simulink model "NeuromuscularModel"  (R2019b)
settings: Solver=ode15s  StartTime=0.0  StopTime=inf  MaxStep=.01  RelTol=1e-4  AbsTol=1e-6  EnableMultiTasking=on
values from neighbouring files (symbols this model uses):
  LceOffsetTA = 1-0.5*w    [ControlParams2.m]
  legLengthClr = .9    (= 0.9)    [ControlParams2.m]    (also in assignGains.m = Gains(20); assignGains2.m = Gains(20); assignGainsSagittal.m = GainsSagittal(39))
  LongDelay = 0.020    (= 0.02)    [ControlParams2.m]
  MidDelay = 0.010    (= 0.01)    [ControlParams2.m]
  N = 82    [vcmaes_1.5cm_0.9ms_Umb10_kneelim1_mstoptorque2.mat]
  ShortDelay = 0.005    [ControlParams2.m]
  simbiconGainD = 5*pi/180    (= 0.0872664625997)    [ControlParams2.m]    (also in assignGains.m = Gains(21); assignGains2.m = Gains(21); assignGainsSagittal.m = GainsSagittal(41))
  simbiconGainDAbd = 0.1421    [ControlParams2.m]    (also in assignGains.m = Gains(33))
  simbiconGainV = 5*pi/180    (= 0.0872664625997)    [ControlParams2.m]    (also in assignGains.m = Gains(22); assignGains2.m = Gains(22); assignGainsSagittal.m = GainsSagittal(42))
  simbiconGainVAbd = 0.2148    [ControlParams2.m]    (also in assignGains.m = Gains(34))
  simbiconLegAngle0 = 85*pi/180    (= 1.4835298642)    [ControlParams2.m]    (also in assignGains.m = Gains(23); assignGains2.m = Gains(23); assignGainsSagittal.m = GainsSagittal(40))
  simbiconLegAngle0Abd = -0.0133    [ControlParams2.m]    (also in assignGains.m = Gains(32))
undefined symbols (not defined in the file or in its folder): footCenterToCGDist, footInertia, footMass, g, hatHipToCenterDistLen, loptGAS, loptTA, lslackGAS, magnitude, phimaxGASa, phimaxGASk, phirefGASa, phirefGASk, rGASa, rGASk, rhoGASa, rhoGASk, X, Y, Z
libraries: NeuroMuscularLibrary x101, nesl_utility x30, sm_lib x21, simulink x4, simulink_extras x2, NeuroMuscularLibrary2 x2
(part 3 of 3)

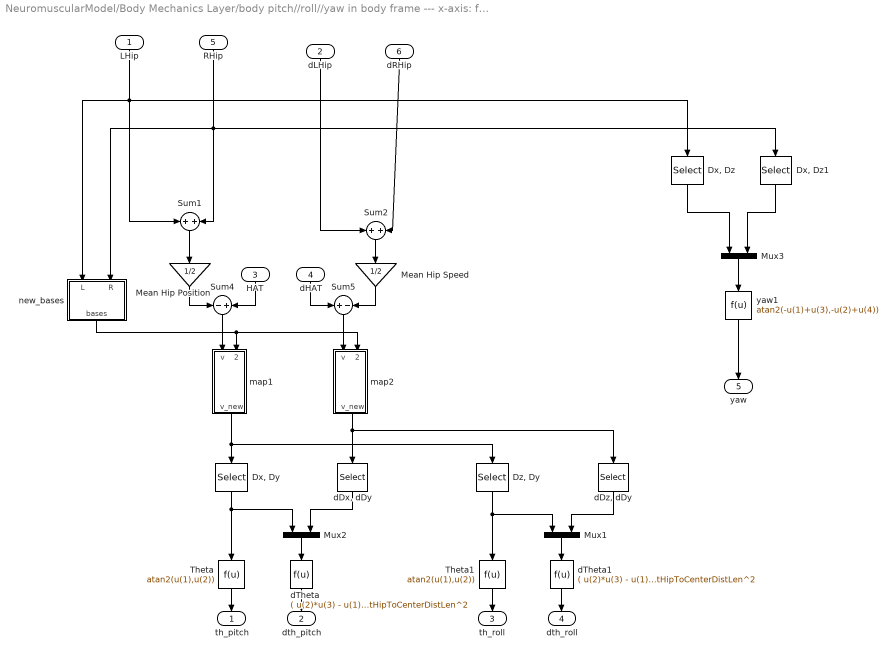
== system NeuromuscularModel/Body Mechanics Layer/body pitch//roll//yaw in body frame --- x-axis: forward y-axis: leftward z-axis: parallel to gravity ==
  LHip : Inport
  dLHip : Inport  Port=2
  HAT : Inport  Port=3
  dHAT : Inport  Port=4
  RHip : Inport  Port=5
  dRHip : Inport  Port=6
  " Mean Hip Speed" : Gain  Gain=1/2
  "Dx, Dy" : Selector  InputPortWidth=3  IndexOptions=Index vector (dialog)  Indices=[1 2]  OutputSizes=1
  "Dx, Dz" : Selector  InputPortWidth=3  IndexOptions=Index vector (dialog)  Indices=[1 3]  OutputSizes=1
  "Dx, Dz1" : Selector  InputPortWidth=3  IndexOptions=Index vector (dialog)  Indices=[1 3]  OutputSizes=1
  "Dz, Dy" : Selector  InputPortWidth=3  IndexOptions=Index vector (dialog)  Indices=[3 2]  OutputSizes=1
  Mean Hip Position : Gain  Gain=1/2
  Mux1 : Mux  Inputs=2
  Mux2 : Mux  Inputs=2
  Mux3 : Mux  Inputs=2
  Sum1 : Sum
  Sum2 : Sum
  Sum4 : Sum  Inputs=-+
  Sum5 : Sum  Inputs=+-
  Theta : Fcn  Expr=atan2(u(1),u(2))
  Theta1 : Fcn  Expr=atan2(u(1),u(2))
  "dDx, dDy" : Selector  InputPortWidth=3  IndexOptions=Index vector (dialog)  Indices=[1 2]  OutputSizes=1
  "dDz, dDy" : Selector  InputPortWidth=3  IndexOptions=Index vector (dialog)  Indices=[3 2]  OutputSizes=1
  dTheta : Fcn  Expr=( u(2)*u(3) - u(1)*u(4) ) / hatHipToCenterDistLen^2
  dTheta1 : Fcn  Expr=( u(2)*u(3) - u(1)*u(4) ) / hatHipToCenterDistLen^2
  map1 : Subsystem
  map2 : Subsystem
  new_bases : Subsystem
  yaw1 : Fcn  Expr=atan2(-u(1)+u(3),-u(2)+u(4))
  th_pitch : Outport
  dth_pitch : Outport  Port=2
  th_roll : Outport  Port=3
  dth_roll : Outport  Port=4
  yaw : Outport  Port=5
  wires:
  dHAT/1 -> Sum5/1
  "dDx, dDy"/1 -> Mux2/2
  Mux2/1 -> dTheta/1
  Sum1/1 -> Mean Hip Position/1
  Sum2/1 -> " Mean Hip Speed"/1
  HAT/1 -> Sum4/2
  Mean Hip Position/1 -> Sum4/1
  " Mean Hip Speed"/1 -> Sum5/2
  "Dx, Dy"/1 -> Mux2/1, Theta/1
  LHip/1 -> Sum1/1, new_bases/1(L), "Dx, Dz"/1
  RHip/1 -> Sum1/2, new_bases/2(R), "Dx, Dz1"/1
  dLHip/1 -> Sum2/1
  dRHip/1 -> Sum2/2
  Theta/1 -> th_pitch/1
  dTheta/1 -> dth_pitch/1
  Sum4/1 -> map1/1(v)
  map1/1(v_new) -> "Dx, Dy"/1, "Dz, Dy"/1
  new_bases/1(bases) -> map1/2(basis), map2/2(basis)
  Sum5/1 -> map2/1(v)
  map2/1(v_new) -> "dDx, dDy"/1, "dDz, dDy"/1
  "dDz, dDy"/1 -> Mux1/2
  Mux1/1 -> dTheta1/1
  "Dz, Dy"/1 -> Mux1/1, Theta1/1
  Theta1/1 -> th_roll/1
  dTheta1/1 -> dth_roll/1
  "Dx, Dz"/1 -> Mux3/1
  "Dx, Dz1"/1 -> Mux3/2
  Mux3/1 -> yaw1/1
  yaw1/1 -> yaw/1

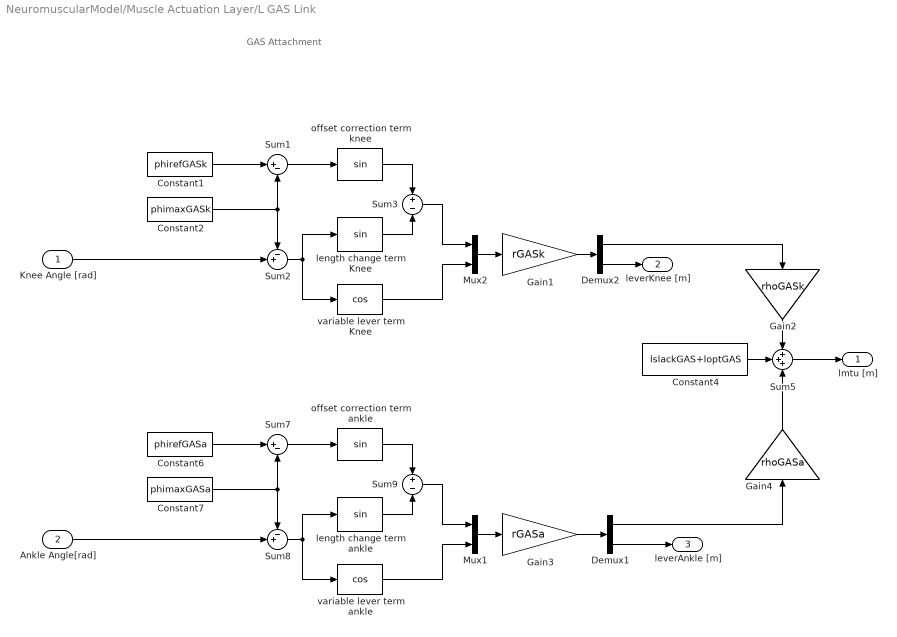
== system NeuromuscularModel/Muscle Actuation Layer/L GAS Link ==
  note: GAS Attachment
  Knee Angle [rad] : Inport
  Ankle Angle[rad] : Inport  Port=2
  Constant1 : Constant  Value=phirefGASk
  Constant2 : Constant  Value=phimaxGASk
  Constant4 : Constant  Value=lslackGAS+loptGAS
  Constant6 : Constant  Value=phirefGASa
  Constant7 : Constant  Value=phimaxGASa
  Demux1 : Demux  Outputs=2
  Demux2 : Demux  Outputs=2
  Gain1 : Gain  Gain=rGASk
  Gain2 : Gain  Gain=rhoGASk
  Gain3 : Gain  Gain=rGASa
  Gain4 : Gain  Gain=rhoGASa
  Mux1 : Mux  Inputs=2
  Mux2 : Mux  Inputs=2
  Sum1 : Sum  Inputs=|+-
  Sum2 : Sum  Inputs=-+|
  Sum3 : Sum  Inputs=+-
  Sum5 : Sum  Inputs=+++
  Sum7 : Sum  Inputs=|+-
  Sum8 : Sum  Inputs=-+|
  Sum9 : Sum  Inputs=+-
  length change term Knee : Trigonometry
  length change term ankle : Trigonometry
  offset correction term ankle : Trigonometry
  offset correction term knee : Trigonometry
  variable lever term Knee : Trigonometry  Operator=cos
  variable lever term ankle : Trigonometry  Operator=cos
  lmtu [m] : Outport
  leverKnee [m] : Outport  Port=2
  leverAnkle [m] : Outport  Port=3
  wires:
  Ankle Angle[rad]/1 -> Sum8/2
  Sum5/1 -> lmtu [m]/1
  variable lever term ankle/1 -> Mux1/2
  Demux1/2 -> leverAnkle [m]/1
  Sum8/1 -> variable lever term ankle/1, length change term ankle/1
  Constant7/1 -> Sum8/1, Sum7/2
  Sum7/1 -> offset correction term ankle/1
  Constant6/1 -> Sum7/1
  length change term ankle/1 -> Sum9/2
  offset correction term ankle/1 -> Sum9/1
  Sum9/1 -> Mux1/1
  Constant4/1 -> Sum5/2
  Mux1/1 -> Gain3/1
  Gain3/1 -> Demux1/1
  Demux1/1 -> Gain4/1
  Gain4/1 -> Sum5/3
  Knee Angle [rad]/1 -> Sum2/2
  variable lever term Knee/1 -> Mux2/2
  Sum2/1 -> variable lever term Knee/1, length change term Knee/1
  Constant2/1 -> Sum2/1, Sum1/2
  Sum1/1 -> offset correction term knee/1
  Constant1/1 -> Sum1/1
  length change term Knee/1 -> Sum3/2
  offset correction term knee/1 -> Sum3/1
  Sum3/1 -> Mux2/1
  Mux2/1 -> Gain1/1
  Gain1/1 -> Demux2/1
  Demux2/2 -> leverKnee [m]/1
  Demux2/1 -> Gain2/1
  Gain2/1 -> Sum5/1

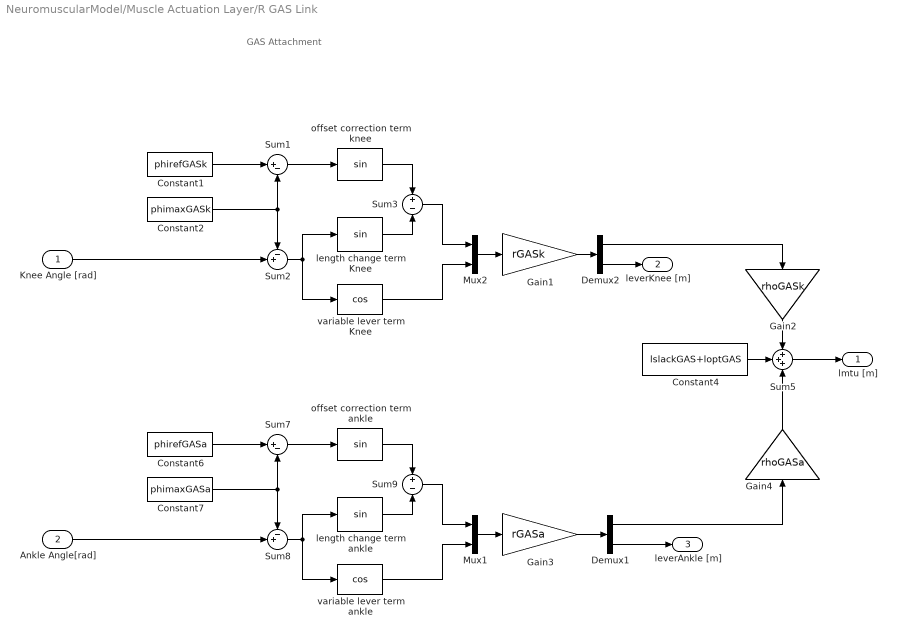
== system NeuromuscularModel/Muscle Actuation Layer/R GAS Link ==
  note: GAS Attachment
  Knee Angle [rad] : Inport
  Ankle Angle[rad] : Inport  Port=2
  Constant1 : Constant  Value=phirefGASk
  Constant2 : Constant  Value=phimaxGASk
  Constant4 : Constant  Value=lslackGAS+loptGAS
  Constant6 : Constant  Value=phirefGASa
  Constant7 : Constant  Value=phimaxGASa
  Demux1 : Demux  Outputs=2
  Demux2 : Demux  Outputs=2
  Gain1 : Gain  Gain=rGASk
  Gain2 : Gain  Gain=rhoGASk
  Gain3 : Gain  Gain=rGASa
  Gain4 : Gain  Gain=rhoGASa
  Mux1 : Mux  Inputs=2
  Mux2 : Mux  Inputs=2
  Sum1 : Sum  Inputs=|+-
  Sum2 : Sum  Inputs=-+|
  Sum3 : Sum  Inputs=+-
  Sum5 : Sum  Inputs=+++
  Sum7 : Sum  Inputs=|+-
  Sum8 : Sum  Inputs=-+|
  Sum9 : Sum  Inputs=+-
  length change term Knee : Trigonometry
  length change term ankle : Trigonometry
  offset correction term ankle : Trigonometry
  offset correction term knee : Trigonometry
  variable lever term Knee : Trigonometry  Operator=cos
  variable lever term ankle : Trigonometry  Operator=cos
  lmtu [m] : Outport
  leverKnee [m] : Outport  Port=2
  leverAnkle [m] : Outport  Port=3
  wires:
  Ankle Angle[rad]/1 -> Sum8/2
  Sum5/1 -> lmtu [m]/1
  variable lever term ankle/1 -> Mux1/2
  Demux1/2 -> leverAnkle [m]/1
  Sum8/1 -> variable lever term ankle/1, length change term ankle/1
  Constant7/1 -> Sum8/1, Sum7/2
  Sum7/1 -> offset correction term ankle/1
  Constant6/1 -> Sum7/1
  length change term ankle/1 -> Sum9/2
  offset correction term ankle/1 -> Sum9/1
  Sum9/1 -> Mux1/1
  Constant4/1 -> Sum5/2
  Mux1/1 -> Gain3/1
  Gain3/1 -> Demux1/1
  Demux1/1 -> Gain4/1
  Gain4/1 -> Sum5/3
  Knee Angle [rad]/1 -> Sum2/2
  variable lever term Knee/1 -> Mux2/2
  Sum2/1 -> variable lever term Knee/1, length change term Knee/1
  Constant2/1 -> Sum2/1, Sum1/2
  Sum1/1 -> offset correction term knee/1
  Constant1/1 -> Sum1/1
  length change term Knee/1 -> Sum3/2
  offset correction term knee/1 -> Sum3/1
  Sum3/1 -> Mux2/1
  Mux2/1 -> Gain1/1
  Gain1/1 -> Demux2/1
  Demux2/2 -> leverKnee [m]/1
  Demux2/1 -> Gain2/1
  Gain2/1 -> Sum5/1

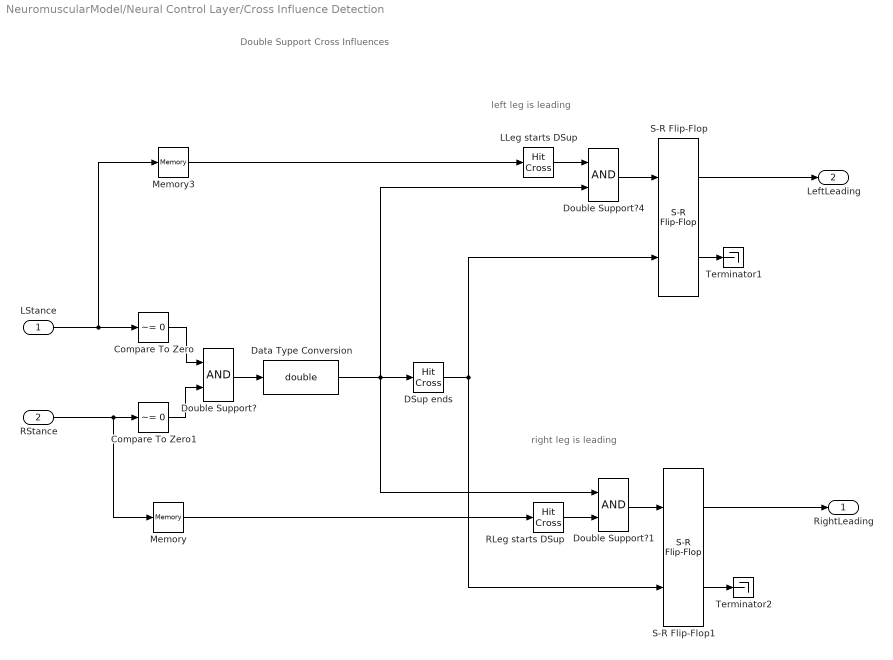
== system NeuromuscularModel/Neural Control Layer/Cross Influence Detection ==
  note: right leg is leading
  note: left leg is leading
  note: Double Support Cross Influences
  LStance : Inport
  RStance : Inport  Port=2
  Compare To Zero : simulink/Logic and Bit Operations/Compare To Zero  relop=~=  OutDataTypeStr=boolean
  Compare To Zero1 : simulink/Logic and Bit Operations/Compare To Zero  relop=~=  OutDataTypeStr=boolean
  DSup ends : HitCross  HitCrossingOffset=0.5  HitCrossingDirection=falling  ZeroCross=off
  Data Type Conversion : DataTypeConversion  OutDataTypeStr=double
  Double Support? : Logic  AllPortsSameDT=off
  Double Support?1 : Logic  AllPortsSameDT=off
  Double Support?4 : Logic  AllPortsSameDT=off
  LLeg starts DSup : HitCross  HitCrossingOffset=0.5  HitCrossingDirection=rising  ZeroCross=off
  Memory : Memory
  Memory3 : Memory
  RLeg starts DSup : HitCross  HitCrossingOffset=0.5  HitCrossingDirection=rising  ZeroCross=off
  S-R Flip-Flop : simulink_extras/Flip Flops/S-R Flip-Flop  initial_condition=0
  S-R Flip-Flop1 : simulink_extras/Flip Flops/S-R Flip-Flop  initial_condition=0
  Terminator1 : Terminator
  Terminator2 : Terminator
  RightLeading : Outport
  LeftLeading : Outport  Port=2
  wires:
  S-R Flip-Flop/2 -> Terminator1/1
  S-R Flip-Flop/1 -> LeftLeading/1
  S-R Flip-Flop1/2 -> Terminator2/1
  LStance/1 -> Memory3/1, Compare To Zero/1
  RStance/1 -> Compare To Zero1/1, Memory/1
  S-R Flip-Flop1/1 -> RightLeading/1
  Memory/1 -> RLeg starts DSup/1
  RLeg starts DSup/1 -> Double Support?1/2
  Double Support?1/1 -> S-R Flip-Flop1/1
  Memory3/1 -> LLeg starts DSup/1
  LLeg starts DSup/1 -> Double Support?4/1
  Double Support?4/1 -> S-R Flip-Flop/1
  DSup ends/1 -> S-R Flip-Flop/2, S-R Flip-Flop1/2
  Compare To Zero/1 -> Double Support?/1
  Compare To Zero1/1 -> Double Support?/2
  Double Support?/1 -> Data Type Conversion/1
  Data Type Conversion/1 -> Double Support?1/1, Double Support?4/2, DSup ends/1

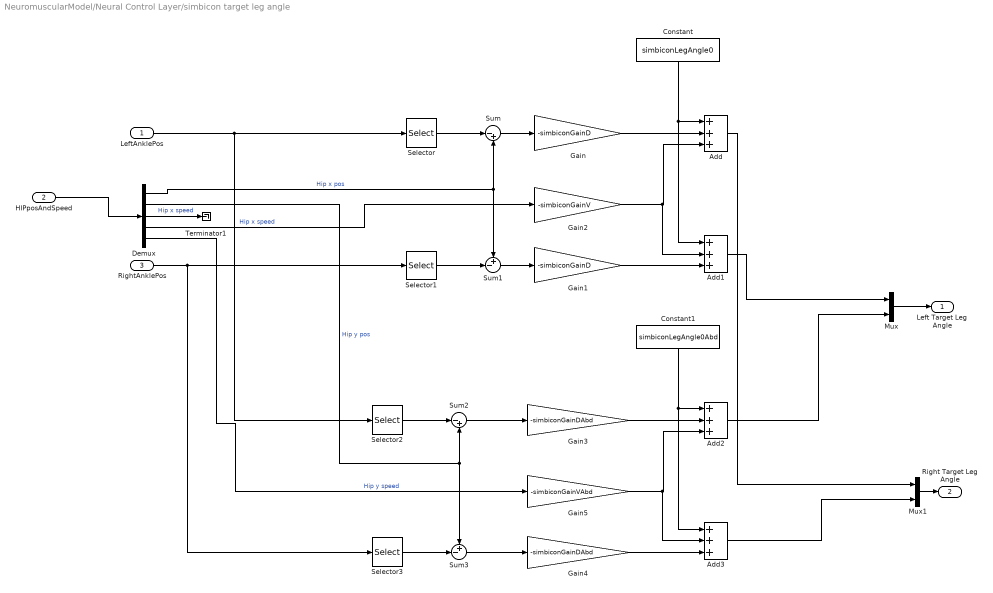
== system NeuromuscularModel/Neural Control Layer/simbicon target leg angle ==
  LeftAnklePos : Inport
  HIPposAndSpeed : Inport  Port=2
  RightAnklePos : Inport  Port=3
  Add{,1..3} (4 alike) : Sum  Inputs=+++
  Constant : Constant  Value=simbiconLegAngle0
  Constant1 : Constant  Value=simbiconLegAngle0Abd
  Demux : Demux  Outputs=5
  Gain : Gain  Gain=-simbiconGainD
  Gain1 : Gain  Gain=-simbiconGainD
  Gain2 : Gain  Gain=-simbiconGainV
  Gain3 : Gain  Gain=-simbiconGainDAbd
  Gain4 : Gain  Gain=-simbiconGainDAbd
  Gain5 : Gain  Gain=-simbiconGainVAbd
  Mux : Mux  Inputs=2
  Mux1 : Mux  Inputs=2
  Selector : Selector  InputPortWidth=3  IndexOptions=Index vector (dialog)  Indices=[1]  OutputSizes=1
  Selector1 : Selector  InputPortWidth=3  IndexOptions=Index vector (dialog)  Indices=[1]  OutputSizes=1
  Selector2 : Selector  InputPortWidth=3  IndexOptions=Index vector (dialog)  Indices=[3]  OutputSizes=1
  Selector3 : Selector  InputPortWidth=3  IndexOptions=Index vector (dialog)  Indices=3  OutputSizes=1
  Sum : Sum  Inputs=|-+
  Sum1 : Sum  Inputs=+-|
  Sum2 : Sum  Inputs=|-+
  Sum3 : Sum  Inputs=+-|
  Terminator1 : Terminator
  Left Target Leg Angle : Outport
  Right Target Leg Angle : Outport  Port=2
  wires:
  HIPposAndSpeed/1 -> Demux/1
  Demux/1 -> Sum/2, Sum1/1  "Hip x pos"
  Sum/1 -> Gain/1
  Sum1/1 -> Gain1/1
  Gain/1 -> Add/2
  Gain2/1 -> Add1/2, Add/3
  Gain1/1 -> Add1/3
  Constant/1 -> Add/1, Add1/1
  LeftAnklePos/1 -> Selector2/1, Selector/1
  Selector/1 -> Sum/1
  RightAnklePos/1 -> Selector3/1, Selector1/1
  Selector1/1 -> Sum1/2
  Demux/2 -> Sum2/2, Sum3/1  "Hip y pos"
  Selector3/1 -> Sum3/2
  Gain5/1 -> Add3/2, Add2/3
  Selector2/1 -> Sum2/1
  Gain4/1 -> Add3/3
  Sum2/1 -> Gain3/1
  Gain3/1 -> Add2/2
  Sum3/1 -> Gain4/1
  Constant1/1 -> Add2/1, Add3/1
  Demux/4 -> Gain2/1  "Hip x speed"
  Demux/5 -> Gain5/1  "Hip y speed"
  Demux/3 -> Terminator1/1  "Hip x speed"
  Add1/1 -> Mux/1
  Add2/1 -> Mux/2
  Add3/1 -> Mux1/2
  Add/1 -> Mux1/1
  Mux1/1 -> Right Target Leg Angle/1
  Mux/1 -> Left Target Leg Angle/1

== system NeuromuscularModel/Body Mechanics Layer/body pitch//roll//yaw in body frame --- x-axis: forward y-axis: leftward z-axis: parallel to gravity/map1 ==
  v : Inport
  basis : Inport  Port=2
  Demux : Demux  Outputs=3
  Dot Product : DotProduct  InputSameDT=on  OutDataTypeStr=Inherit: Inherit via internal rule
  Dot Product1 : DotProduct  InputSameDT=on  OutDataTypeStr=Inherit: Inherit via internal rule
  Dot Product2 : DotProduct  InputSameDT=on  OutDataTypeStr=Inherit: Inherit via internal rule
  Mux3 : Mux  Inputs=3
  v_new : Outport
  wires:
  v/1 -> Dot Product2/2, Dot Product1/2, Dot Product/2
  Dot Product/1 -> Mux3/1
  Dot Product1/1 -> Mux3/2
  Dot Product2/1 -> Mux3/3
  Mux3/1 -> v_new/1  "v1"
  basis/1 -> Demux/1
  Demux/1 -> Dot Product/1
  Demux/2 -> Dot Product1/1
  Demux/3 -> Dot Product2/1

== system NeuromuscularModel/Body Mechanics Layer/body pitch//roll//yaw in body frame --- x-axis: forward y-axis: leftward z-axis: parallel to gravity/map2 ==
  v : Inport
  basis : Inport  Port=2
  Demux : Demux  Outputs=3
  Dot Product : DotProduct  InputSameDT=on  OutDataTypeStr=Inherit: Inherit via internal rule
  Dot Product1 : DotProduct  InputSameDT=on  OutDataTypeStr=Inherit: Inherit via internal rule
  Dot Product2 : DotProduct  InputSameDT=on  OutDataTypeStr=Inherit: Inherit via internal rule
  Mux3 : Mux  Inputs=3
  v_new : Outport
  wires:
  v/1 -> Dot Product2/2, Dot Product1/2, Dot Product/2
  Dot Product/1 -> Mux3/1
  Dot Product1/1 -> Mux3/2
  Dot Product2/1 -> Mux3/3
  Mux3/1 -> v_new/1  "v1"
  basis/1 -> Demux/1
  Demux/1 -> Dot Product/1
  Demux/2 -> Dot Product1/1
  Demux/3 -> Dot Product2/1

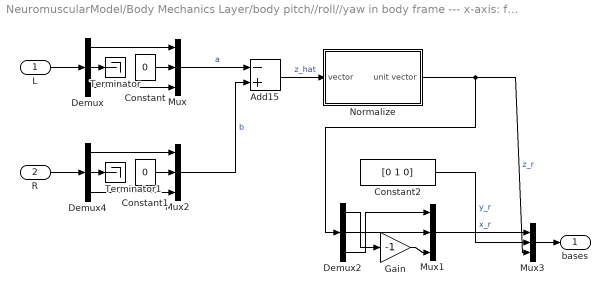
== system NeuromuscularModel/Body Mechanics Layer/body pitch//roll//yaw in body frame --- x-axis: forward y-axis: leftward z-axis: parallel to gravity/new_bases ==
  L : Inport
  R : Inport  Port=2
  Add15 : Sum  Inputs=-+
  Constant : Constant  Value=0
  Constant1 : Constant  Value=0
  Constant2 : Constant  Value=[0 1 0]
  Demux : Demux  Outputs=3
  Demux2 : Demux  Outputs=3
  Demux4 : Demux  Outputs=3
  Gain : Gain  Gain=-1
  Mux{,1..3} (4 alike) : Mux  Inputs=3
  Normalize : Subsystem
  Terminator : Terminator
  Terminator1 : Terminator
  bases : Outport
  wires:
  Constant2/1 -> Mux3/2  "y_r"
  Demux2/1 -> Gain/1
  Demux2/3 -> Mux1/1
  Demux2/2 -> Mux1/2
  Add15/1 -> Normalize/1(vector)  "z_hat"
  Normalize/1(unit vector) -> Demux2/1, Mux3/3  "z_r"
  Mux2/1 -> Add15/2  "b"
  Demux4/2 -> Terminator1/1
  Constant1/1 -> Mux2/2
  Demux4/3 -> Mux2/3
  Demux4/1 -> Mux2/1
  Mux/1 -> Add15/1  "a"
  Demux/2 -> Terminator/1
  Constant/1 -> Mux/2
  Demux/3 -> Mux/3
  Demux/1 -> Mux/1
  L/1 -> Demux/1
  R/1 -> Demux4/1
  Mux3/1 -> bases/1
  Gain/1 -> Mux1/3
  Mux1/1 -> Mux3/1  "x_r"

== system NeuromuscularModel/Body Mechanics Layer/body pitch//roll//yaw in body frame --- x-axis: forward y-axis: leftward z-axis: parallel to gravity/new_bases/Normalize ==
  vector : Inport
  Constant1 : Constant  Value=.5
  Math Function : Math  Operator=magnitude^2  SaturateOnIntegerOverflow=on
  Product : Product  Inputs=*/  RndMeth=Zero
  Sqrt : Math  Operator=pow  OutputSignalType=real  SaturateOnIntegerOverflow=on
  Sum of Elements : Sum  Inputs=+
  unit vector : Outport
  wires:
  Sqrt/1 -> Product/2
  Sum of Elements/1 -> Sqrt/1
  Math Function/1 -> Sum of Elements/1
  vector/1 -> Product/1, Math Function/1
  Product/1 -> unit vector/1  "x_r"
  Constant1/1 -> Sqrt/2
